simulink model "DCmotormodel"  (Simulink 7.7)
settings: Solver=ode45  StartTime=0.0  StopTime=15  RelTol=1e-3
values from neighbouring files (symbols this model uses):
  J = 0.02    [DCmotor.m]    (also in constantes_robot.m)
  Kb = 0.1    [DCmotor.m]    (also in constantes_robot.m)
  Kf = 0.2    [DCmotor.m]    (also in constantes_robot.m)
  Kff = 1/dcgain(dcm(1))    [DCmotor.m]    (also in constantes_robot.m)
  Km = 0.1    [DCmotor.m]    (also in constantes_robot.m)
  L = 0.5    [DCmotor.m]    (also in constantes_robot.m)
  R = 2.0    (= 2)    [DCmotor.m]    (also in constantes_robot.m)
settings Model: Creator=Ángel  LastModifiedBy=Ángel

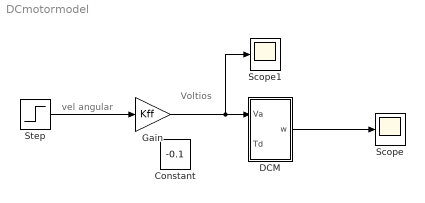
== system DCmotormodel ==
  note: Voltios
  note: vel angular
  Constant : Constant  Value=-0.1
  DCM : Subsystem
  Gain : Gain  Gain=Kff
  Scope : Scope
  Scope1 : Scope
  Step : Step  Time=0  SampleTime=0
  wires:
  Gain/1 -> DCM/1(Va), Scope1/1
  DCM/1(w) -> Scope/1
  Step/1 -> Gain/1

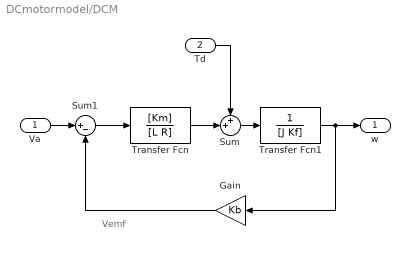
== system DCmotormodel/DCM ==
  note: Vemf
  Va : Inport
  Td : Inport  Port=2
  Gain : Gain  Gain=Kb
  Sum : Sum  Inputs=++|
  Sum1 : Sum  Inputs=|+-
  Transfer Fcn : TransferFcn  Numerator=[Km]  Denominator=[L R]
  Transfer Fcn1 : TransferFcn  Denominator=[J Kf]
  w : Outport
  wires:
  Transfer Fcn/1 -> Sum/2
  Gain/1 -> Sum1/2
  Sum1/1 -> Transfer Fcn/1
  Sum/1 -> Transfer Fcn1/1
  Transfer Fcn1/1 -> Gain/1, w/1
  Td/1 -> Sum/1
  Va/1 -> Sum1/1
